simulink subsystem "InjectorNHNE"  (R2020b)
settings: Solver=VariableStepAuto  StartTime=0.0  StopTime=10.0  RelTol=1e-3
model mask{dischargeCoeff=0.8, numHolesPort1=5, numHolesPort2=5, holeAreaPort1=2e-5, holeAreaPort2=2e-5}
  mask prompts: dischargeCoeff "Cd"; numHolesPort1 "Number of holes port 1"; numHolesPort2 "Number of holes port 2"; holeAreaPort1 "Single hole area port 1 (m^2)"; holeAreaPort2 "Single hole area port 2 (m^2)"
libraries: nesl_utility x3, fl_lib x3, SimscapeCustomBlocks_lib x2
settings Model: Creator=Edward  LastModifiedBy=Edward

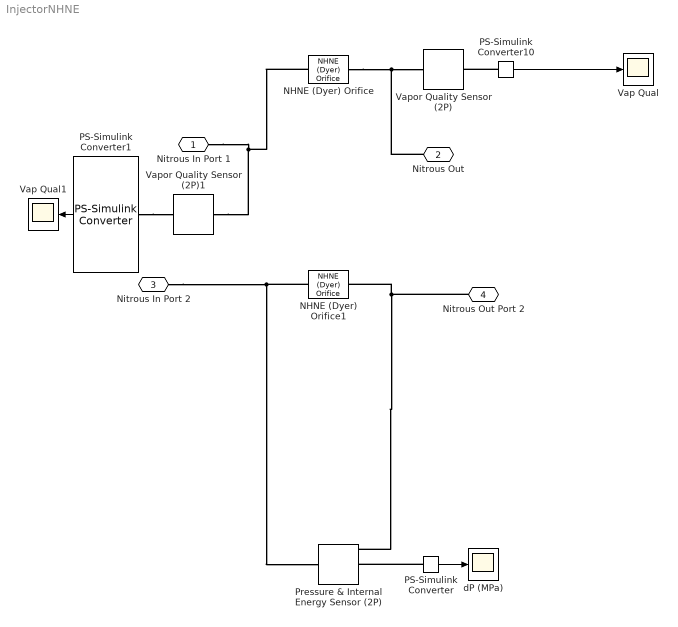
== system InjectorNHNE ==
  NHNE (Dyer) Orifice : SimscapeCustomBlocks_lib/NHNE (Dyer) Orifice  area=Sim.preInjectorPipe.crossSection m^2  orifice_area=numHolesPort1 * holeAreaPort1 m^2  Cd=dischargeCoeff
      settings: InternalSimscapePortConfiguration="{\"Bottom\":[],\"Left\":[{\"id\":\"A\",\"label\":\"A\",\"type\":\"foundation.two_phase_fluid.two_phase_fluid\"}],\"Right\":[{\"id\":\"B\",\"label\":\"B\",\"type\":\"foundation.two_phase_fluid.two_phase_fluid\"}],\"Top\":[]}"
  NHNE (Dyer) Orifice1 : SimscapeCustomBlocks_lib/NHNE (Dyer) Orifice  area=Sim.preInjectorPipe.crossSection m^2  orifice_area=numHolesPort2 * holeAreaPort2 m^2  Cd=dischargeCoeff
      settings: InternalSimscapePortConfiguration="{\"Bottom\":[],\"Left\":[{\"id\":\"A\",\"label\":\"A\",\"type\":\"foundation.two_phase_fluid.two_phase_fluid\"}],\"Right\":[{\"id\":\"B\",\"label\":\"B\",\"type\":\"foundation.two_phase_fluid.two_phase_fluid\"}],\"Top\":[]}"
  PS-Simulink Converter : nesl_utility/PS-Simulink Converter  PhysicalDomain=network_engine_domain  SubClassName=ps_output  LeftPortType=input  RightPortType=output  PseudoPeriodic=off  Frequencies=[]  Unit=inherit  AffineConversion=off
  PS-Simulink Converter1 : nesl_utility/PS-Simulink Converter  PhysicalDomain=network_engine_domain  SubClassName=ps_output  LeftPortType=input  RightPortType=output  PseudoPeriodic=off  Frequencies=[]  Unit=inherit  AffineConversion=off
  PS-Simulink Converter10 : nesl_utility/PS-Simulink Converter  PhysicalDomain=network_engine_domain  SubClassName=ps_output  LeftPortType=input  RightPortType=output  PseudoPeriodic=off  Frequencies=[]  Unit=inherit  AffineConversion=off
  Pressure & Internal Energy Sensor (2P) : fl_lib/Two-Phase Fluid/Sensors/Pressure & Internal Energy Sensor (2P)
      settings: SourceProductBaseCode=SS  InternalSimscapePortConfiguration="{\"Bottom\":[],\"Left\":[{\"id\":\"A\",\"label\":\"A\",\"type\":\"foundation.two_phase_fluid.two_phase_fluid\"}],\"Right\":[{\"id\":\"B\",\"label\":\"B\",\"type\":\"foundation.two_phase_fluid.two_phase_fluid\"},{\"id\":\"P\",\"label\":\"P\",\"type\":\"output\"},{\"id\":\"U\",\"label\":\"U\",\"type\":\"output\"}],\"Top\":[]}"
  Vap Qual : Scope
  Vap Qual1 : Scope
  Vapor Quality Sensor (2P) : fl_lib/Two-Phase Fluid/Sensors/Vapor Quality Sensor (2P)  vapor_fraction_spec=foundation.enum.vapor_fraction_spec.quality
      settings: SourceProductBaseCode=SS  InternalSimscapePortConfiguration="{\"Bottom\":[],\"Left\":[{\"id\":\"A\",\"label\":\"A\",\"type\":\"foundation.two_phase_fluid.two_phase_fluid\"}],\"Right\":[{\"id\":\"X\",\"label\":\"X\",\"type\":\"output\"}],\"Top\":[]}"
  Vapor Quality Sensor (2P)1 : fl_lib/Two-Phase Fluid/Sensors/Vapor Quality Sensor (2P)  vapor_fraction_spec=foundation.enum.vapor_fraction_spec.quality
      settings: SourceProductBaseCode=SS  InternalSimscapePortConfiguration="{\"Bottom\":[],\"Left\":[{\"id\":\"A\",\"label\":\"A\",\"type\":\"foundation.two_phase_fluid.two_phase_fluid\"}],\"Right\":[{\"id\":\"X\",\"label\":\"X\",\"type\":\"output\"}],\"Top\":[]}"
  dP (MPa) : Scope
  Nitrous In Port 1 : PMIOPort  Side=Left
  Nitrous Out : PMIOPort  Port=2  Side=Right
  Nitrous In Port 2 : PMIOPort  Port=3  Side=Left
  Nitrous Out Port 2 : PMIOPort  Port=4  Side=Right
  wires:
  PS-Simulink Converter/1 -> dP (MPa)/1
  PS-Simulink Converter10/1 -> Vap Qual/1
  PS-Simulink Converter1/1 -> Vap Qual1/1
  connections:
  Nitrous Out/RConn1 -- NHNE (Dyer) Orifice/RConn1 -- Vapor Quality Sensor (2P)/LConn1
  Vapor Quality Sensor (2P)1/LConn1 -- NHNE (Dyer) Orifice/LConn1 -- Nitrous In Port 1/RConn1
  Nitrous In Port 2/RConn1 -- NHNE (Dyer) Orifice1/LConn1 -- Pressure & Internal Energy Sensor (2P)/LConn1
  Nitrous Out Port 2/RConn1 -- NHNE (Dyer) Orifice1/RConn1 -- Pressure & Internal Energy Sensor (2P)/RConn1
  PS-Simulink Converter/LConn1 -- Pressure & Internal Energy Sensor (2P)/RConn2
  PS-Simulink Converter10/LConn1 -- Vapor Quality Sensor (2P)/RConn1
  PS-Simulink Converter1/LConn1 -- Vapor Quality Sensor (2P)1/RConn1
